simulink model "explicit_force"  (R2017a)
settings: Solver=FixedStepDiscrete  StartTime=0.0  StopTime=inf  RelTol=1e-3  EnableMultiTasking=on
undefined symbols (not defined in the file or in its folder): DiscIntNeverNeededParam, Down, GPTRIP1SEL, GPTRIP2SEL, PWM_Counter_Period, TZ1, TZ2, Up
libraries: dspsigops x3, c280xlib x2, c2802xlib x2, c2806xlib x2, simulink x1, dspsrcs4 x1
settings Model: ExtModeTrigDuration=10  Creator=Kalman  LastModifiedBy=ata.otaran
settings DataIOCC: LimitDataPoints=on  SaveFormat=Array
settings OptimizationCC: LifeSpan=Inf  MaxStackSize=512
settings DebuggingCC: AllowSymbolicDim=off  SFUnexpectedBacktrackingDiag=warning  SFNoUnconditionalDefaultTransitionDiag=warning  SFExecutionAtInitializationDiag=none
settings HardwareCC: ProdBitPerChar=16  ProdBitPerInt=16  ProdBitPerPointer=16  ProdBitPerSizeT=32  ProdBitPerPtrDiffT=32  ProdLargestAtomicInteger=Integer  ProdLargestAtomicFloat=None  ProdWordSize=16  ProdLongLongMode=on  ProdHWDeviceType=Texas Instruments->C2000
settings ModelReferenceCC: PropagateSignalLabelsOutOfModel=off
settings SFSimCC: MATLABDynamicMemAlloc=off
settings RTWCC: SystemTargetFile=ert.tlc  HardwareBoard=TI Piccolo F2806x  TLCOptions=-aInlineSetEventsForThisBaseRateFcn=TLC_FALSE -aSuppressMultiTaskScheduler=TLC_FALSE -aRateBasedStepFcn=1  TemplateMakefile=ert_default_tmf  Description=Embedded Coder  Toolchain=Texas Instruments Code Composer Studio v5 (C2000)
settings CodeAppCC: IgnoreCustomStorageClasses=off
settings ERTTargetCC: CodeReplacementLibrary=TI C28x  MultiwordLength=2048  ConvertIfToSwitch=off  SuppressUnreachableDefaultCases=off
settings ConfigComp: CovMetricSettings=dw  CovHtmlReporting=on  CovSaveCumulativeToWorkspaceVar=on  CovSaveSingleToWorkspaceVar=on  CovExternalEMLEnable=off

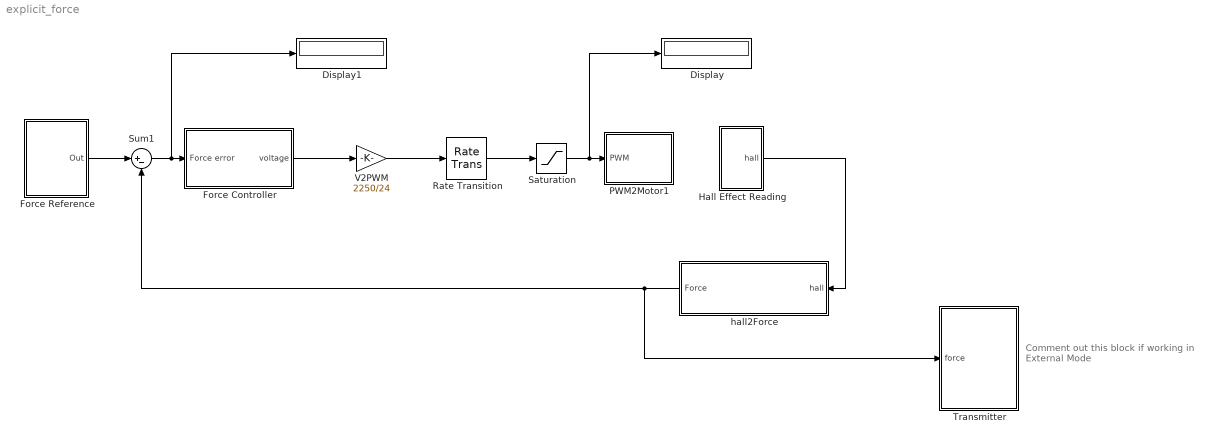
== system explicit_force ==
  note: Comment out this block if
      | working in External Mode
  Display : Display
  Display1 : Display
  Force Controller : Subsystem
  Force Reference : Subsystem
  Hall Effect Reading : Subsystem
  PWM2Motor1 : Subsystem
  Rate Transition : RateTransition
  Saturation : Saturate  UpperLimit=2250  LowerLimit=-2250
  Sum1 : Sum  Inputs=|+-
  Transmitter : Subsystem
  V2PWM : Gain  Gain=2250/24
  hall2Force : Subsystem
  wires:
  Saturation/1 -> Display/1, PWM2Motor1/1(PWM)
  Force Reference/1(Out) -> Sum1/1
  Rate Transition/1 -> Saturation/1
  Hall Effect Reading/1(hall) -> hall2Force/1(hall)
  Force Controller/1(voltage) -> V2PWM/1
  Sum1/1 -> Display1/1, Force Controller/1(Force error)
  V2PWM/1 -> Rate Transition/1
  hall2Force/1(Force) -> Sum1/2, Transmitter/1(force)

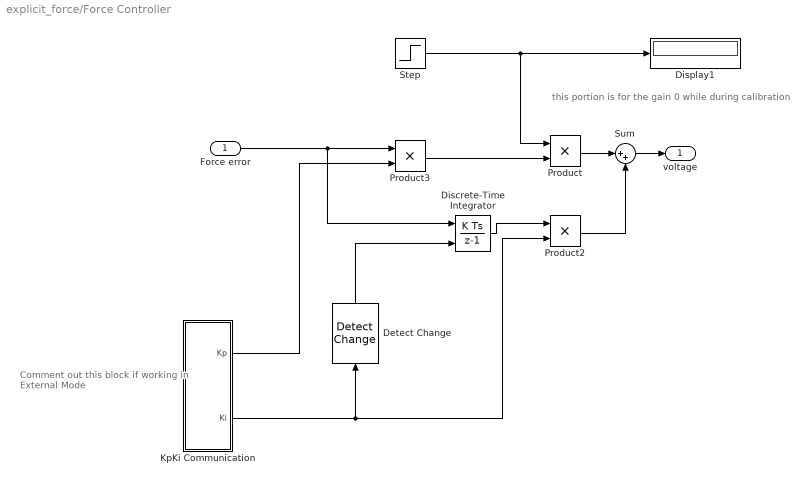
== system explicit_force/Force Controller ==
  note: this portion is for the gain 0 while during calibration
  note: Comment out this block if
      | working in External Mode
  Force error : Inport
  Detect Change : simulink/Logic and Bit Operations/Detect Change  vinit=0  OutDataTypeStr=boolean
  Discrete-Time Integrator : DiscreteIntegrator  ExternalReset=rising  InitialConditionSetting=State (most efficient)  SampleTime=-1  ICPrevOutput=DiscIntNeverNeededParam  ICPrevScaledInput=DiscIntNeverNeededParam
  Display1 : Display
  KpKi Communication : Subsystem
  Product : Product
  Product2 : Product
  Product3 : Product
  Step : Step  Time=0.2
  Sum : Sum  Inputs=|++
  voltage : Outport
  wires:
  Product/1 -> Sum/1
  Product3/1 -> Product/2
  Step/1 -> Product/1, Display1/1
  Discrete-Time Integrator/1 -> Product2/1
  KpKi Communication/1(Kp) -> Product3/2
  Sum/1 -> voltage/1
  Product2/1 -> Sum/2
  KpKi Communication/2(Ki) -> Product2/2, Detect Change/1
  Detect Change/1 -> Discrete-Time Integrator/2
  Force error/1 -> Discrete-Time Integrator/1, Product3/1

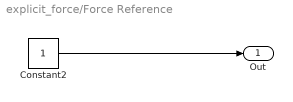
== system explicit_force/Force Reference ==
  Constant2 : Constant
  Out : Outport
  wires:
  Constant2/1 -> Out/1

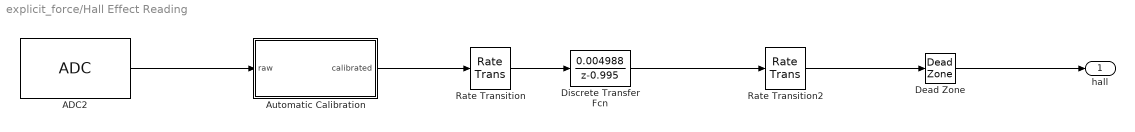
== system explicit_force/Hall Effect Reading ==
  ADC2 : c2802xlib/ADC  ADCModule=1  samplingMode=Single sample mode  ADCResolution=12-bit (Single-ended input)  useSOC1=SOC1  useSOC2=SOC0_SOC1  SOCAcquisitionWindow=7  SOCTriggerSource=Software  SOCInterruptTrigger=No ADCINT  Ts=-1  dType=int32  postInterrupt=off  interruptSel=ADCINT1  ADCINTContinuous=off  endma=off  chdma=1  blkParamProc=C2000  conv1=ADCINA7  conv2=ADCINA7 and ADCINB7  conv1_Type4=ADCIN0  conv2_Type4=ADCIN0 and ADCIN1
      settings: SourceProductName=Embedded Coder Support Package for Texas Instruments C2000 Processors
  Automatic Calibration : Subsystem
  Dead Zone : DeadZone  LowerValue=-3  UpperValue=3  SaturateOnIntegerOverflow=on
  Discrete Transfer Fcn : DiscreteTransferFcn  Numerator=[0.004988]  Denominator=[1 -0.995]
  Rate Transition : RateTransition
  Rate Transition2 : RateTransition  OutPortSampleTime=0.001
  hall : Outport
  wires:
  Discrete Transfer Fcn/1 -> Rate Transition2/1
  Rate Transition/1 -> Discrete Transfer Fcn/1
  Dead Zone/1 -> hall/1
  Rate Transition2/1 -> Dead Zone/1
  Automatic Calibration/1(calibrated) -> Rate Transition/1
  ADC2/1 -> Automatic Calibration/1(raw)

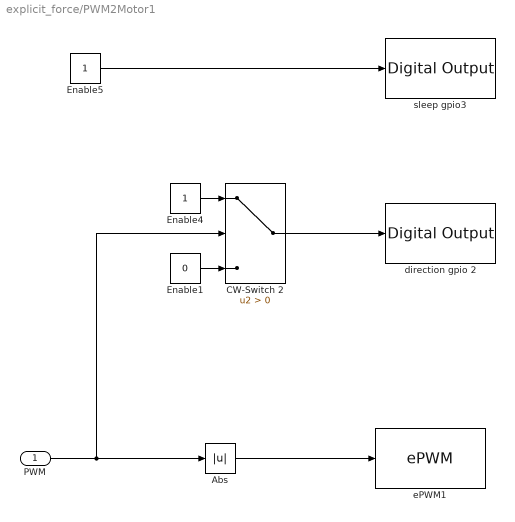
== system explicit_force/PWM2Motor1 ==
  PWM : Inport
  Abs : Abs
  CW-Switch 2 : Switch  Criteria=u2 > Threshold
  Enable1 : Constant  Value=0
  Enable4 : Constant
  Enable5 : Constant
  direction gpio 2 : c2806xlib/Digital Output  GPIO_Number=GPIO0~GPIO7  GPIO_Bit0=off  GPIO_BIT0_Toggle=off  GPIO_Bit1=off  GPIO_BIT1_Toggle=off  GPIO_Bit2=on  GPIO_BIT2_Toggle=off  GPIO_Bit3=off  GPIO_BIT3_Toggle=off  GPIO_Bit4=off  GPIO_BIT4_Toggle=off  GPIO_Bit5=off  GPIO_BIT5_Toggle=off  GPIO_Bit6=off  GPIO_BIT6_Toggle=off  GPIO_Bit7=off  GPIO_BIT7_Toggle=off
      settings: SourceProductName=Embedded Coder Support Package for Texas Instruments C2000 Processors  SourceProductBaseCode=TIC2000
  ePWM1 : c2802xlib/ePWM  useModule=ePWM1  ePWMxLINKTBPRD=Not Linked  periodUnits=Clock cycles  timerSource=Specify via dialog  timerPeriod_clk=PWM_Counter_Period+1  timerPeriod_sec=0.0001  tbshadow=Counter equals to zero  countingMode=Up-Down  phaseActiveEnable=Disable  phaseDirection=Count down after sync  phaseActive=0  synchronizationEnable=off  dcaevt1Sync=off  dcbevt1Sync=off  synchronizationOption=Disable  clockPrescale=1  HSclockPrescale=1  enswap=off  ePWMxAStatus=on  ePWMxAactionLogic1=Do nothing  ePWMxAactionLogic2=Do nothing  ePWMxAactionLogic3=Clear  ePWMxAactionLogic4=Set  ePWMxAactionLogic5=Do nothing  ePWMxAactionLogic6=Do nothing  ePWMxALoadMode=Load on counter equals to zero (CTR=Zero)  ePWMxACSFenable=off  ePWMxACSFvalue=Forcing disable  ePWMxASFreload=Zero  ePWMxBStatus=off  ePWMxBactionLogic1=Set  ePWMxBactionLogic2=Clear  ePWMxBactionLogic3=Do nothing  ePWMxBactionLogic4=Do nothing  ePWMxBactionLogic5=Clear  ePWMxBactionLogic6=Set  ePWMxBLoadMode=Load on counter equals to zero (CTR=Zero)  ePWMxBCSFenable=off  ePWMxBCSFvalue=Forcing disable  ePWMxBSFreload=Zero  ePWNxBOutWay=off  ePWMxLINKCMPA=Not Linked  CMPAUnits=Clock cycles  CMPASource=Input port  CMPAValue_per=50  CMPAValue_clk=PWM_Counter_Period/2+1  enCMPAshadow=Counter equals to zero  ePWMxLINKCMPB=Not Linked  CMPBUnits=Clock cycles  CMPBSource=Specify via dialog  CMPBValue_per=50  CMPBValue_clk=PWM_Counter_Period/2+1  enCMPBshadow=Counter equals to zero  ePWMxLINKCMPC=Not Linked  CMPCUnits=Clock cycles  CMPCSource=Specify via dialog  CMPCValue_per=50  CMPCValue_clk=32000  enCMPCshadow=Counter equals to zero  ePWMxLINKCMPD=Not Linked  CMPDUnits=Clock cycles  CMPDSource=Specify via dialog  CMPDValue_per=50  CMPDValue_clk=32000  enCMPDshadow=Counter equals to zero  enableDBePWMxA=off  enableDBePWMxB=off  enhalfcycle=off  DBpolarity=Active high (AH)  DBedgeDelay=Positive  DBSource_ePWMxA=ePWMxA  DBSource_ePWMxB=ePWMxA  DBperiodSource=Specify via dialog  REDperiod=0  FEDperiod=0  adcstartModuleA=off  adcrequestEventA=First event  adcstartEventA=Digital Compare Module A Event 1 start of conversion (DCAEVT1.soc)  adcstartEventA_type2=Digital Compare Module A Event 1 start of conversion (DCAEVT1.soc)  adcstartModuleB=off  adcrequestEventB=First event  adcstartEventB=Counter equals to zero (CTR=Zero)  adcstartEventB_type2=Counter equals to zero (CTR=Zero)  intEn=off  intPrd=First event  intSel=Counter equals to zero (CTR=Zero)  intSel_type2=Counter equals to zero (CTR=Zero)  hrpe=off  enHRPWM=off  HRPWM_LoadMode=Counter equals to period (CTR=PRD)  HRPWM_CTLMode=Duty or Period control mode  HRPWM_EDGMode=Both edge  hrpeb=off  enHRPWMB=off  HRPWM_LoadModeB=Counter equals to zero (CTR=ZERO)  HRPWM_CTLModeB=Duty or Period control mode  HRPWM_EDGModeB=Both edge  enSFO=on  enautoconv=on  chopperEnable=off  chopperFrequency=1  chopperFirstwidth=1  chopperDuty=12.5%  tripZonesource=Specify via dialog  tzselOSHT1=off  tzselOSHT2=off  tzselOSHT3=off  tzselOSHDCAEV1=off  tzselOSHDCBEV1=off  tzselCBC1=off  tzselCBC2=off  tzselCBC3=off  tzselCBCDCAEV2=off  tzselCBCDCBEV2=off  tzselOSHT4=off  tzselOSHT5=off  tzselOSHT6=off  tzselCBC4=off  tzselCBC5=off  tzselCBC6=off  enTzOstIntr=off  enTzCbcIntr=off  enTzDCAEVT1Intr=off  enTzDCAEVT2Intr=off  enTzDCBEVT1Intr=off  enTzDCBEVT2Intr=off  ePWMxAforced=No action  ePWMxBforced=No action  DCAEVT1forced=No action  DCBEVT1forced=No action  DCAEVT2forced=No action  DCBEVT2forced=No action  dcah=Trip Zone 1 input (TZ1)  dcal=Trip Zone 2 input (TZ2)  dcbh=Trip Zone 1 input (TZ1)  dcbl=Trip Zone 2 input (TZ2)  dcah_type2=GPTRIP1SEL/(TZ1)  dcal_type2=GPTRIP2SEL/(TZ2)  dcbh_type2=GPTRIP1SEL/(TZ1)  dcbl_type2=GPTRIP2SEL/(TZ2)  gendcaevt1=Event disabled  gendcaevt2=Event disabled  gendcbevt1=Event disabled  gendcbevt2=Event disabled  dcaevt1src=DCAEVT1 with sync  dcaevt2src=DCAEVT2 with sync  dcbevt1src=DCBEVT1 with sync  dcbevt2src=DCBEVT2 with sync  pulsesel=Counter equals to zero (CTR=Zero)  blankinv=off  blankoffset=0  blankwidth=0  evsrcsel=Filtered version of DCAEVT1 (DCAEVT1FILT)  encape=off  PwmType=C2000
      settings: SourceProductName=Embedded Coder Support Package for Texas Instruments C2000 Processors
  sleep gpio3 : c2806xlib/Digital Output  GPIO_Number=GPIO0~GPIO7  GPIO_Bit0=off  GPIO_BIT0_Toggle=off  GPIO_Bit1=off  GPIO_BIT1_Toggle=off  GPIO_Bit2=off  GPIO_BIT2_Toggle=off  GPIO_Bit3=on  GPIO_BIT3_Toggle=off  GPIO_Bit4=off  GPIO_BIT4_Toggle=off  GPIO_Bit5=off  GPIO_BIT5_Toggle=off  GPIO_Bit6=off  GPIO_BIT6_Toggle=off  GPIO_Bit7=off  GPIO_BIT7_Toggle=off
      settings: SourceProductName=Embedded Coder Support Package for Texas Instruments C2000 Processors  SourceProductBaseCode=TIC2000
  wires:
  PWM/1 -> Abs/1, CW-Switch 2/2
  Enable1/1 -> CW-Switch 2/3
  Enable4/1 -> CW-Switch 2/1
  Enable5/1 -> sleep gpio3/1
  CW-Switch 2/1 -> direction gpio 2/1
  Abs/1 -> ePWM1/1

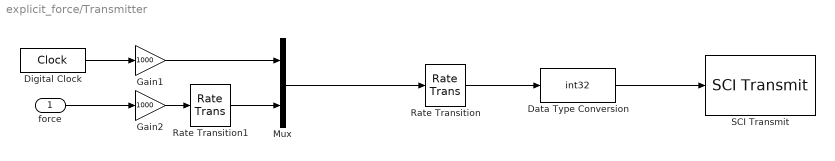
== system explicit_force/Transmitter ==
  force : Inport
  Data Type Conversion : DataTypeConversion  OutDataTypeStr=int32  ConvertRealWorld=Stored Integer (SI)
  Digital Clock : DigitalClock  SampleTime=0.0001
  Gain1 : Gain  Gain=1000
  Gain2 : Gain  Gain=1000
  Mux : Mux  Inputs=2
  Rate Transition : RateTransition  Integrity=off  OutPortSampleTime=0.02
  Rate Transition1 : RateTransition  Integrity=off  OutPortSampleTime=0.0001
  SCI Transmit : c280xlib/SCI Transmit  sciModule=A  dataHead='S'  dataTail='E'  postInterrupt=on  numFifo=3
      settings: SourceProductName=Embedded Coder Support Package for Texas Instruments C2000 Processors
  wires:
  Rate Transition/1 -> Data Type Conversion/1
  Data Type Conversion/1 -> SCI Transmit/1
  Digital Clock/1 -> Gain1/1
  force/1 -> Gain2/1
  Gain1/1 -> Mux/1
  Gain2/1 -> Rate Transition1/1
  Mux/1 -> Rate Transition/1
  Rate Transition1/1 -> Mux/2

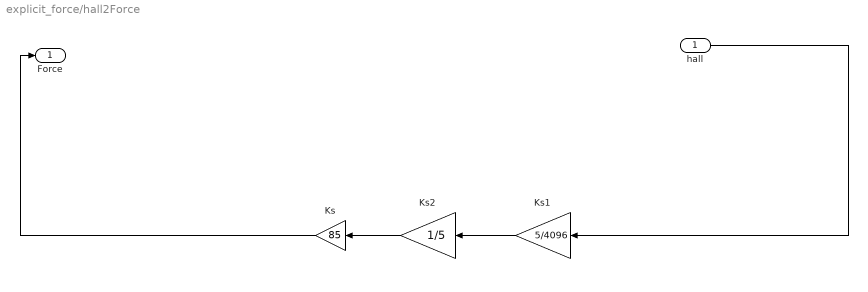
== system explicit_force/hall2Force ==
  hall : Inport
  Ks : Gain  Gain=85
  Ks1 : Gain  Gain=5/4096
  Ks2 : Gain  Gain=1/5
  Force : Outport
  wires:
  hall/1 -> Ks1/1
  Ks1/1 -> Ks2/1
  Ks2/1 -> Ks/1
  Ks/1 -> Force/1

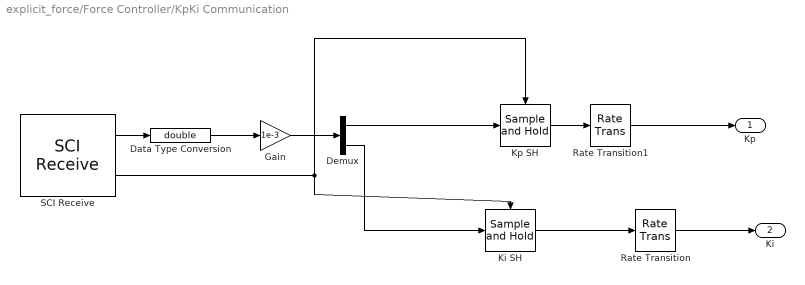
== system explicit_force/Force Controller/KpKi Communication ==
  Data Type Conversion : DataTypeConversion  OutDataTypeStr=double
  Demux : Demux  Outputs=2
  Gain : Gain  Gain=1e-3
  Ki SH : dspsigops/Sample and Hold  trig=Rising edge  initCond=0  latchinput=off
  Kp SH : dspsigops/Sample and Hold  trig=Rising edge  initCond=0  latchinput=off
  Rate Transition : RateTransition
  Rate Transition1 : RateTransition
  SCI Receive : c280xlib/SCI Receive  sciModule=A  dataHead='S'  dataTail='E'  dataType=int32  dataDim=2  initValue=0  errOption=Output the last received value  errValue=0  sampleTime=0.05  outputStatus=on  postInterrupt=off  numFifo=1
      settings: SourceProductName=Embedded Coder Support Package for Texas Instruments C2000 Processors  SourceProductBaseCode=TIC2000
  Kp : Outport
  Ki : Outport  Port=2
  wires:
  Demux/2 -> Ki SH/1
  SCI Receive/1 -> Data Type Conversion/1
  Rate Transition1/1 -> Kp/1
  Rate Transition/1 -> Ki/1
  SCI Receive/2 -> Kp SH/Trigger, Ki SH/Trigger
  Data Type Conversion/1 -> Gain/1
  Kp SH/1 -> Rate Transition1/1
  Demux/1 -> Kp SH/1
  Ki SH/1 -> Rate Transition/1
  Gain/1 -> Demux/1

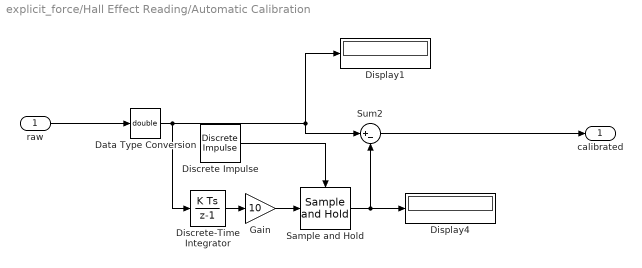
== system explicit_force/Hall Effect Reading/Automatic Calibration ==
  raw : Inport
  Data Type Conversion : DataTypeConversion  OutDataTypeStr=double
  Discrete Impulse : dspsrcs4/Discrete  Impulse  Delay=1000  SampleTime=-1  FrameSample=1  OutputFrames=off  dataType=double  isSigned=on  wordLen=16  udDataType=sfix(16)  fracBitsMode=Best precision  numFracBits=15  OutDataTypeStr=double  LastOutDataTypeStr=double
  Discrete-Time Integrator : DiscreteIntegrator  InitialConditionSetting=State (most efficient)  SampleTime=0.0001  ICPrevOutput=DiscIntNeverNeededParam  ICPrevScaledInput=DiscIntNeverNeededParam
  Display1 : Display
  Display4 : Display
  Gain : Gain  Gain=10
  Sample and Hold : dspsigops/Sample and Hold  trig=Rising edge  initCond=0  latchinput=off
  Sum2 : Sum  Inputs=|+-
  calibrated : Outport
  wires:
  raw/1 -> Data Type Conversion/1
  Discrete Impulse/1 -> Sample and Hold/Trigger
  Data Type Conversion/1 -> Discrete-Time Integrator/1, Sum2/1, Display1/1
  Sample and Hold/1 -> Display4/1, Sum2/2
  Discrete-Time Integrator/1 -> Gain/1
  Gain/1 -> Sample and Hold/1
  Sum2/1 -> calibrated/1
